simulink model "nominal_tracking"  (R2020b)
settings: Solver=ode45  StartTime=0.0  StopTime=5  RelTol=1e-3
undefined symbols (not defined in the file or in its folder): Beq_hat, daq, degs2rpm, denH1, drv, gbox, Jeq_hat, mot, N_u, N_x, numH1, rads2rpm, rpm2rads, sens, step_size, tau_hat
settings Model: Creator=utente  LastModifiedBy=giuli
settings DataIOCC: ReturnWorkspaceOutputs=off

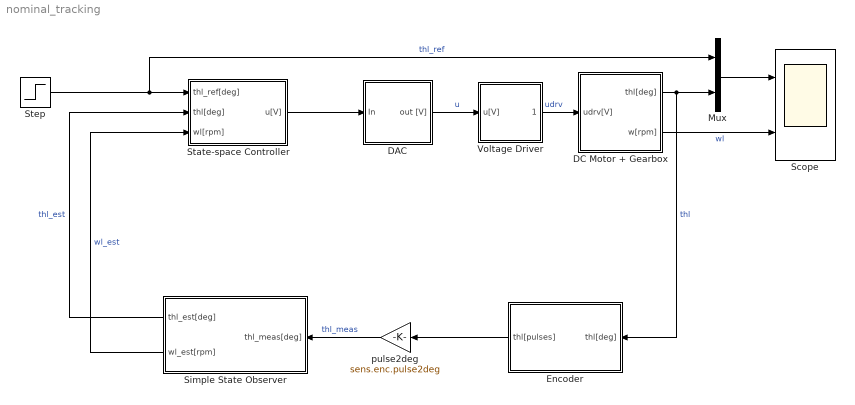
== system nominal_tracking ==
  DAC : Subsystem
  DC Motor + Gearbox : Subsystem
  Encoder : Subsystem
  Mux : Mux  Inputs=2
  Scope : Scope  NumInputPorts=2
  Simple State Observer : Subsystem
  State-space Controller : Subsystem
  Step : Step  After=step_size  SampleTime=0
  Voltage Driver : Subsystem
  pulse2deg : Gain  Gain=sens.enc.pulse2deg
  wires:
  State-space Controller/1(u[V]) -> DAC/1(In)
  DAC/1(out [V]) -> Voltage Driver/1(u[V])  "u"
  Voltage Driver/1(udrv[V]) -> DC Motor + Gearbox/1(udrv[V])  "udrv"
  Encoder/1(thl[pulses]) -> pulse2deg/1
  DC Motor + Gearbox/1(thl[deg]) -> Mux/2, Encoder/1(thl[deg])  "thl"
  DC Motor + Gearbox/2(w[rpm]) -> Scope/2  "wl"
  Step/1 -> Mux/1, State-space Controller/1(thl_ref[deg])  "thl_ref"
  pulse2deg/1 -> Simple State Observer/1(thl_meas[deg])  "thl_meas"
  Simple State Observer/1(thl_est[deg]) -> State-space Controller/2(thl[deg])  "thl_est"
  Simple State Observer/2(wl_est[rpm]) -> State-space Controller/3(wl[rpm])  "wl_est"
  Mux/1 -> Scope/1

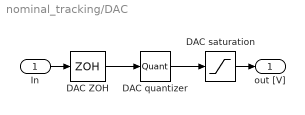
== system nominal_tracking/DAC ==
  In : Inport
  DAC quantizer : Quantizer  QuantizationInterval=daq.dac.q
  DAC saturation : Saturate  UpperLimit=daq.dac.fs  LowerLimit=-daq.dac.fs
  DAC ZOH : ZeroOrderHold  SampleTime=0.001
  out [V] : Outport
  wires:
  DAC ZOH/1 -> DAC quantizer/1
  DAC quantizer/1 -> DAC saturation/1
  In/1 -> DAC ZOH/1
  DAC saturation/1 -> out [V]/1

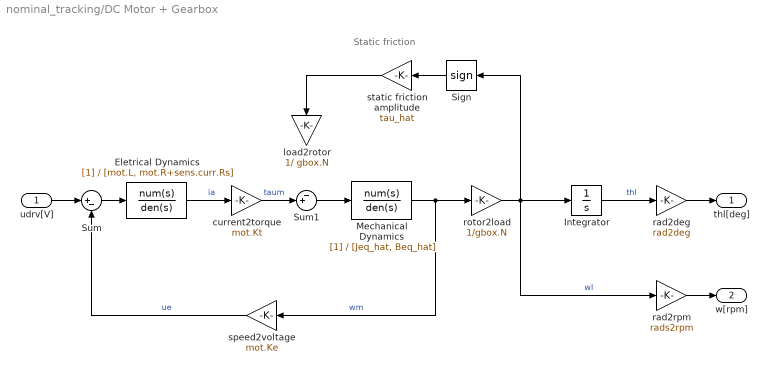
== system nominal_tracking/DC Motor + Gearbox ==
  note: Static friction
  udrv[V] : Inport
  Eletrical Dynamics : TransferFcn  Denominator=[mot.L, mot.R+sens.curr.Rs]
  Integrator : Integrator
  Mechanical Dynamics : TransferFcn  Denominator=[Jeq_hat, Beq_hat]
  Sign : Signum  ZeroCross=off
  Sum : Sum  Inputs=|+-
  Sum1 : Sum  Inputs=-+|
  current2torque : Gain  Gain=mot.Kt
  load2rotor : Gain  Gain=1/ gbox.N
  rad2deg : Gain  Gain=rad2deg
  "rad2rpm " : Gain  Gain=rads2rpm
  rotor2load : Gain  Gain=1/gbox.N
  speed2voltage : Gain  Gain=mot.Ke
  static friction amplitude : Gain  Gain=tau_hat
  thl[deg] : Outport  VectorParamsAs1DForOutWhenUnconnected=off
  w[rpm] : Outport  Port=2  VectorParamsAs1DForOutWhenUnconnected=off
  wires:
  Eletrical Dynamics/1 -> current2torque/1  "ia"
  udrv[V]/1 -> Sum/1
  Sum/1 -> Eletrical Dynamics/1
  current2torque/1 -> Sum1/2  "taum"
  Sum1/1 -> Mechanical Dynamics/1
  Mechanical Dynamics/1 -> rotor2load/1, speed2voltage/1  "wm"
  rotor2load/1 -> Integrator/1, "rad2rpm "/1, Sign/1  "wl"
  Integrator/1 -> rad2deg/1  "thl"
  rad2deg/1 -> thl[deg]/1
  "rad2rpm "/1 -> w[rpm]/1
  static friction amplitude/1 -> load2rotor/1
  Sign/1 -> static friction amplitude/1
  speed2voltage/1 -> Sum/2  "ue"

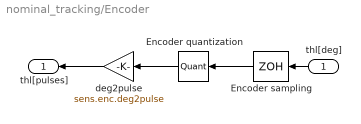
== system nominal_tracking/Encoder ==
  thl[deg] : Inport
  Encoder quantization : Quantizer  QuantizationInterval=sens.enc.pulse2deg
  Encoder sampling : ZeroOrderHold  SampleTime=-1
  deg2pulse : Gain  Gain=sens.enc.deg2pulse
  thl[pulses] : Outport
  wires:
  thl[deg]/1 -> Encoder sampling/1
  Encoder quantization/1 -> deg2pulse/1
  Encoder sampling/1 -> Encoder quantization/1
  deg2pulse/1 -> thl[pulses]/1

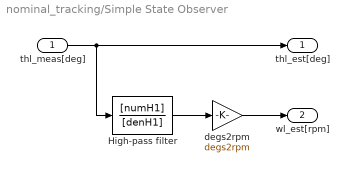
== system nominal_tracking/Simple State Observer ==
  thl_meas[deg] : Inport
  High-pass filter : TransferFcn  Numerator=[numH1]  Denominator=[denH1]
  degs2rpm : Gain  Gain=degs2rpm
  thl_est[deg] : Outport
  wl_est[rpm] : Outport  Port=2
  wires:
  thl_meas[deg]/1 -> thl_est[deg]/1, High-pass filter/1
  High-pass filter/1 -> degs2rpm/1
  degs2rpm/1 -> wl_est[rpm]/1

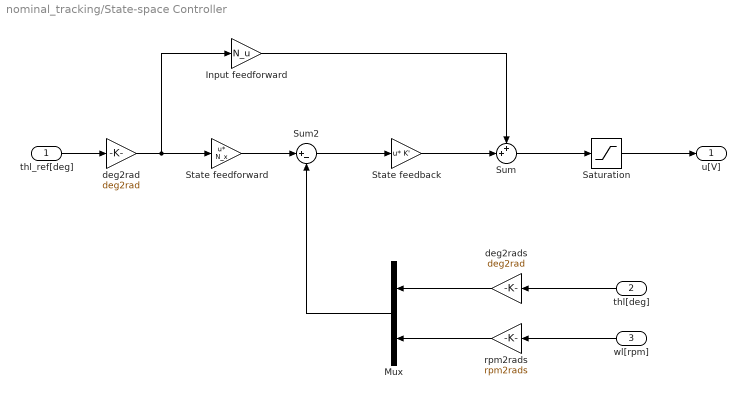
== system nominal_tracking/State-space Controller ==
  thl_ref[deg] : Inport
  thl[deg] : Inport  Port=2
  wl[rpm] : Inport  Port=3
  Input feedforward : Gain  Gain=N_u
  Mux : Mux  Inputs=2
  Saturation : Saturate  UpperLimit=10  LowerLimit=-10
  State feedback : Gain  Gain=K'  Multiplication=Matrix(u*K)
  "State feedforward\t" : Gain  Gain=N_x  Multiplication=Matrix(u*K)
  Sum : Sum  Inputs=++|
  Sum2 : Sum  Inputs=|+-
  deg2rad : Gain  Gain=deg2rad
  deg2rads : Gain  Gain=deg2rad
  rpm2rads : Gain  Gain=rpm2rads
  u[V] : Outport
  wires:
  thl_ref[deg]/1 -> deg2rad/1
  deg2rad/1 -> Input feedforward/1, "State feedforward\t"/1
  State feedback/1 -> Sum/2
  "State feedforward\t"/1 -> Sum2/1
  Sum2/1 -> State feedback/1
  Input feedforward/1 -> Sum/1
  Sum/1 -> Saturation/1
  Saturation/1 -> u[V]/1
  deg2rads/1 -> Mux/1
  rpm2rads/1 -> Mux/2
  thl[deg]/1 -> deg2rads/1
  wl[rpm]/1 -> rpm2rads/1
  Mux/1 -> Sum2/2

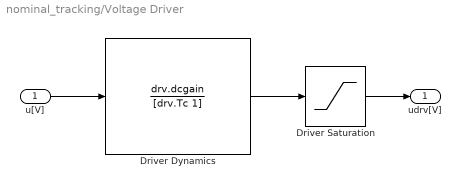
== system nominal_tracking/Voltage Driver ==
  u[V] : Inport
  Driver Dynamics : TransferFcn  Numerator=drv.dcgain  Denominator=[drv.Tc 1]
  Driver Saturation : Saturate  UpperLimit=12  LowerLimit=-12
  udrv[V] : Outport
  wires:
  Driver Dynamics/1 -> Driver Saturation/1
  Driver Saturation/1 -> udrv[V]/1
  u[V]/1 -> Driver Dynamics/1
